simulink model "singlcontact_control_smc_lqr_mydimes_reaction"  (R2024a)
settings: Solver=VariableStepAuto  StartTime=0.0  StopTime=10  FixedStep=0.001  RelTol=1e-3
values from neighbouring files (symbols this model uses):
  ankle_servo_kd = 8    [robotParametersCtrl_mydiem_block_zmp.m]    (also in robotParametersCtrl_quad_modify_mydiem.m; robotParametersCtrl_quad_modify_mydiem_reaction.m)
  ankle_servo_ki = 4    [robotParametersCtrl_mydiem_block_zmp.m]    (also in robotParametersCtrl_quad_modify_mydiem.m; robotParametersCtrl_quad_modify_mydiem_reaction.m)
  ankle_servo_kp = 20    [robotParametersCtrl_mydiem_block_zmp.m]    (also in robotParametersCtrl_quad_modify_mydiem.m; robotParametersCtrl_quad_modify_mydiem_reaction.m)
  deriv_filter_coeff = 100    [robotParametersCtrl_mydiem_block_zmp.m]    (also in robotParametersCtrl_quad_modify_mydiem.m; robotParametersCtrl_quad_modify_mydiem_reaction.m)
  filter_coefficent_pid = 100    [robotParametersCtrl_mydiem_block_zmp.m]    (also in robotParametersCtrl_quad_modify_mydiem.m; robotParametersCtrl_quad_modify_mydiem_reaction.m)
  filter_coefficent_pids = 100    [robotParametersCtrl_quad_modify_mydiem_reaction.m]
  foot_z = 1.5    [robotParametersCtrl_mydiem_block_zmp.m]    (also in robotParametersCtrl_quad_modify_mydiem.m; robotParametersCtrl_quad_modify_mydiem_reaction.m)
  g = 9.81    [ABCDvalues_lqr_quad_mydime_reaction.m]    (also in robotParametersCtrl_mydiem_block_zmp.m = 9.80665; robotParametersCtrl_quad_modify_mydiem.m = 9.80665; robotParametersCtrl_quad_modify_mydiem_reaction.m = 9.80665)
  h = 32    [robotParametersCtrl_mydiem_block_zmp.m]    (also in robotParametersCtrl_quad_modify_mydiem.m; robotParametersCtrl_quad_modify_mydiem_reaction.m)
  height_plane = 0.025    [robotParametersCtrl_mydiem_block_zmp.m]    (also in robotParametersCtrl_quad_modify_mydiem.m; robotParametersCtrl_quad_modify_mydiem_reaction.m)
  hip_pitch_deriv = 20    [robotParametersCtrl_mydiem_block_zmp.m]    (also in robotParametersCtrl_quad_modify_mydiem.m = 200; robotParametersCtrl_quad_modify_mydiem_reaction.m = 200)
  hip_pitch_derivs = 200    [robotParametersCtrl_quad_modify_mydiem_reaction.m]
  hip_pitch_int = 0    [robotParametersCtrl_mydiem_block_zmp.m]    (also in robotParametersCtrl_quad_modify_mydiem.m = 150; robotParametersCtrl_quad_modify_mydiem_reaction.m = 150)
  hip_pitch_ints = 1500    [robotParametersCtrl_quad_modify_mydiem_reaction.m]
  hip_pitch_prop = 10    [robotParametersCtrl_mydiem_block_zmp.m]    (also in robotParametersCtrl_quad_modify_mydiem.m = 500; robotParametersCtrl_quad_modify_mydiem_reaction.m = 500)
  hip_pitch_props = 500    [robotParametersCtrl_quad_modify_mydiem_reaction.m]
  hip_roll_deriv = 28    [robotParametersCtrl_mydiem_block_zmp.m]    (also in robotParametersCtrl_quad_modify_mydiem.m = 280; robotParametersCtrl_quad_modify_mydiem_reaction.m = 280)
  hip_roll_derivs = 280    [robotParametersCtrl_quad_modify_mydiem_reaction.m]
  hip_roll_int = 0    [robotParametersCtrl_mydiem_block_zmp.m]    (also in robotParametersCtrl_quad_modify_mydiem.m = 180; robotParametersCtrl_quad_modify_mydiem_reaction.m = 180)
  hip_roll_ints = 180    [robotParametersCtrl_quad_modify_mydiem_reaction.m]
  hip_roll_prop = 10    [robotParametersCtrl_mydiem_block_zmp.m]    (also in robotParametersCtrl_quad_modify_mydiem.m = 300; robotParametersCtrl_quad_modify_mydiem_reaction.m = 300)
  hip_roll_props = 300    [robotParametersCtrl_quad_modify_mydiem_reaction.m]
  hip_servo_kd = 20    [robotParametersCtrl_mydiem_block_zmp.m]    (also in robotParametersCtrl_quad_modify_mydiem.m; robotParametersCtrl_quad_modify_mydiem_reaction.m)
  hip_servo_ki = 10    [robotParametersCtrl_mydiem_block_zmp.m]    (also in robotParametersCtrl_quad_modify_mydiem.m; robotParametersCtrl_quad_modify_mydiem_reaction.m)
  hip_servo_kp = 60    [robotParametersCtrl_mydiem_block_zmp.m]    (also in robotParametersCtrl_quad_modify_mydiem.m; robotParametersCtrl_quad_modify_mydiem_reaction.m)
  hip_smc_lamda = 85    [robotParametersCtrl_mydiem_block_zmp.m]    (also in robotParametersCtrl_quad_modify_mydiem.m; robotParametersCtrl_quad_modify_mydiem_reaction.m = 95)
  hip_smc_lamdas = 85    [robotParametersCtrl_quad_modify_mydiem_reaction.m]
  hip_smc_new = 25    [robotParametersCtrl_mydiem_block_zmp.m]    (also in robotParametersCtrl_quad_modify_mydiem.m; robotParametersCtrl_quad_modify_mydiem_reaction.m = 45)
  hip_smc_news = 25    [robotParametersCtrl_quad_modify_mydiem_reaction.m]
  init_angs_L = init_angs_R    [robotParametersCtrl_mydiem_block_zmp.m]    (also in robotParametersCtrl_quad_modify_mydiem.m; robotParametersCtrl_quad_modify_mydiem_reaction.m)
  init_angs_R = [0 -sum(init_angs) init_angs(2) 0 init_angs(1)]    [robotParametersCtrl_mydiem_block_zmp.m]    (also in robotParametersCtrl_quad_modify_mydiem.m; robotParametersCtrl_quad_modify_mydiem_reaction.m)
  init_height = h +                torso_z/2 + torso_offset_z + height_plane/2    (= 39.5125)    [robotParametersCtrl_mydiem_block_zmp.m]    (also in robotParametersCtrl_quad_modify_mydiem.m; robotParametersCtrl_quad_modify_mydiem_reaction.m)
  K = lqr(A, B, Q, R)    [ABCDvalues_lqr_quad_mydime_reaction.m]
  knee_pitch_deriv = 10    [robotParametersCtrl_mydiem_block_zmp.m]    (also in robotParametersCtrl_quad_modify_mydiem.m = 100; robotParametersCtrl_quad_modify_mydiem_reaction.m = 100)
  knee_pitch_derivs = 180    [robotParametersCtrl_quad_modify_mydiem_reaction.m]
  knee_pitch_int = 0    [robotParametersCtrl_mydiem_block_zmp.m]    (also in robotParametersCtrl_quad_modify_mydiem.m = 300; robotParametersCtrl_quad_modify_mydiem_reaction.m = 300)
  knee_pitch_ints = 7500    [robotParametersCtrl_quad_modify_mydiem_reaction.m]
  knee_pitch_prop = 10    [robotParametersCtrl_mydiem_block_zmp.m]    (also in robotParametersCtrl_quad_modify_mydiem.m = 400; robotParametersCtrl_quad_modify_mydiem_reaction.m = 400)
  knee_pitch_props = 1200    [robotParametersCtrl_quad_modify_mydiem_reaction.m]
  knee_servo_kd = 10    [robotParametersCtrl_mydiem_block_zmp.m]    (also in robotParametersCtrl_quad_modify_mydiem.m; robotParametersCtrl_quad_modify_mydiem_reaction.m)
  knee_servo_ki = 5    [robotParametersCtrl_mydiem_block_zmp.m]    (also in robotParametersCtrl_quad_modify_mydiem.m; robotParametersCtrl_quad_modify_mydiem_reaction.m)
  knee_servo_kp = 60    [robotParametersCtrl_mydiem_block_zmp.m]    (also in robotParametersCtrl_quad_modify_mydiem.m; robotParametersCtrl_quad_modify_mydiem_reaction.m)
  knee_smc_lamda = 140    [robotParametersCtrl_mydiem_block_zmp.m]    (also in robotParametersCtrl_quad_modify_mydiem.m; robotParametersCtrl_quad_modify_mydiem_reaction.m = 150)
  knee_smc_lamdas = 100    [robotParametersCtrl_quad_modify_mydiem_reaction.m]
  knee_smc_new = 80    [robotParametersCtrl_mydiem_block_zmp.m]    (also in robotParametersCtrl_quad_modify_mydiem.m; robotParametersCtrl_quad_modify_mydiem_reaction.m)
  knee_smc_news = 60    [robotParametersCtrl_quad_modify_mydiem_reaction.m]
  Kwalk = 0.6    [robotParametersCtrl_mydiem_block_zmp.m]    (also in robotParametersCtrl_quad_modify_mydiem.m; robotParametersCtrl_quad_modify_mydiem_reaction.m)
  l1 = 0.20    (= 0.2)    [ABCDvalues_lqr_quad_mydime_reaction.m]
  l2 = 0.20    (= 0.2)    [ABCDvalues_lqr_quad_mydime_reaction.m]
  lower_leg_length = 20    [robotParametersCtrl_mydiem_block_zmp.m]    (also in robotParametersCtrl_quad_modify_mydiem.m; robotParametersCtrl_quad_modify_mydiem_reaction.m)
  m1 = 0.45    [ABCDvalues_lqr_quad_mydime_reaction.m]
  m2 = 0.065    [ABCDvalues_lqr_quad_mydime_reaction.m]
  max_torque = 20    [robotParametersCtrl_mydiem_block_zmp.m]    (also in robotParametersCtrl_quad_modify_mydiem.m; robotParametersCtrl_quad_modify_mydiem_reaction.m)
  motion_time_constant = 0.01    [robotParametersCtrl_mydiem_block_zmp.m]    (also in robotParametersCtrl_quad_modify_mydiem.m; robotParametersCtrl_quad_modify_mydiem_reaction.m)
  plane_x = 25    [robotParametersCtrl_mydiem_block_zmp.m]    (also in robotParametersCtrl_quad_modify_mydiem.m; robotParametersCtrl_quad_modify_mydiem_reaction.m)
  plane_y = 3    [robotParametersCtrl_mydiem_block_zmp.m]    (also in robotParametersCtrl_quad_modify_mydiem.m; robotParametersCtrl_quad_modify_mydiem_reaction.m)
  stepHeight = 0.4    [ABCDvalues_lqr_quad_mydime_reaction.m]
  torso_offset_x = 17    [robotParametersCtrl_mydiem_block_zmp.m]    (also in robotParametersCtrl_quad_modify_mydiem.m; robotParametersCtrl_quad_modify_mydiem_reaction.m)
  torso_offset_x1 = -17    [robotParametersCtrl_mydiem_block_zmp.m]    (also in robotParametersCtrl_quad_modify_mydiem.m; robotParametersCtrl_quad_modify_mydiem_reaction.m)
  torso_offset_z = 0    [robotParametersCtrl_mydiem_block_zmp.m]    (also in robotParametersCtrl_quad_modify_mydiem.m; robotParametersCtrl_quad_modify_mydiem_reaction.m)
  torso_x = 40    [robotParametersCtrl_mydiem_block_zmp.m]    (also in robotParametersCtrl_quad_modify_mydiem.m; robotParametersCtrl_quad_modify_mydiem_reaction.m)
  torso_y = 20    [robotParametersCtrl_mydiem_block_zmp.m]    (also in robotParametersCtrl_quad_modify_mydiem.m; robotParametersCtrl_quad_modify_mydiem_reaction.m)
  torso_z = 15    [robotParametersCtrl_mydiem_block_zmp.m]    (also in robotParametersCtrl_quad_modify_mydiem.m; robotParametersCtrl_quad_modify_mydiem_reaction.m)
  Ts = 0.05    [ABCDvalues_lqr_quad_mydime_reaction.m]
  TsCtrl = 0.05    [robotParametersCtrl_mydiem_block_zmp.m]    (also in robotParametersCtrl_quad_modify_mydiem.m; robotParametersCtrl_quad_modify_mydiem_reaction.m)
  tWalk = 0.3    [robotParametersCtrl_mydiem_block_zmp.m]    (also in robotParametersCtrl_quad_modify_mydiem.m; robotParametersCtrl_quad_modify_mydiem_reaction.m)
  upper_leg_length = 20    [robotParametersCtrl_mydiem_block_zmp.m]    (also in robotParametersCtrl_quad_modify_mydiem.m; robotParametersCtrl_quad_modify_mydiem_reaction.m)
undefined symbols (not defined in the file or in its folder): X, Y, Z
libraries: simulink_extras x256, slpidlib x128, sm_lib x71, simulink x43, nesl_utility x35, walkingRobotUtils x21, dspsrcs4 x18, dspobslib x8
(part 33 of 33)

== system singlcontact_control_smc_lqr_mydimes_reaction/Walking Robot/smc+smcr+neuro1+reaction2/SMC Controllers FR3/Equivalent control/SMC equivalent T1 ==
  theta2 : Inport
  theta1 : Inport  Port=2
  theta2ddot : Inport  Port=3
  theta1dot : Inport  Port=4
  theta2dot : Inport  Port=5
  theta1ddot : Inport  Port=6
  Add{1..4} (4 alike) : Sum
  Add5 : Sum  Inputs=+--+++
  Add6 : Sum  Inputs=++++
  Constant : Constant  Value=0.3
  Constant10 : Constant  Value=m2*l1^2
  Constant11 : Constant  Value=0.3*m1*l1^2
  Constant12 : Constant  Value=m2*l1*l2
  Constant2 : Constant  Value=0.5
  Constant3 : Constant
  Constant4 : Constant  Value=0.5
  Constant5 : Constant
  Constant6 : Constant  Value=g*l1
  Constant7 : Constant  Value=0.5
  Constant9 : Constant  Value=0.3*m2*l2^2
  Cos : Trigonometry  Operator=cos
  Cos1 : Trigonometry  Operator=cos
  Gain1 : Gain  Gain=m2*l2^2
  Gain2 : Gain  Gain=m2*l2*l1
  Gain4 : Gain  Gain=m2*l2*l1
  Gain6 : Gain  Gain=m1
  Gain7 : Gain  Gain=m2
  Gain8 : Gain  Gain=m2*g*l2
  Product{1..3,7..9} (6 alike) : Product
  Product4 : Product  Inputs=4
  Product5 : Product  Inputs=3
  Product6 : Product  Inputs=3
  Sin : Trigonometry
  Sin1 : Trigonometry
  Sin2 : Trigonometry
  Square1 : Math  Operator=square
  T1 : Outport
  wires:
  Add2/1 -> Product1/1
  Product9/1 -> Add2/2
  [lamdaBL1] -> Product9/1
  [edotBL1] -> Product9/2
  Add5/1 -> T1/1
  Product1/1 -> Add5/6
  theta1ddot/1 -> Add2/1
  Add6/1 -> Product1/2
  Product8/1 -> Add6/1
  Constant11/1 -> Add6/2
  Constant10/1 -> Add6/4
  Constant9/1 -> Add6/3
  Cos1/1 -> Product8/1
  Constant12/1 -> Product8/2  "X_dd"
  theta2/1 -> Cos/1, Sin/1, Add4/1, Cos1/1
  Product7/1 -> Add5/5
  Product6/1 -> Add5/4
  Product5/1 -> Add5/3
  Product4/1 -> Add5/2
  Product3/1 -> Add5/1
  Sin2/1 -> Product7/2
  Gain8/1 -> Product7/1
  Add4/1 -> Sin2/1
  Constant7/1 -> Gain8/1
  Constant6/1 -> Product6/3
  Sin1/1 -> Product6/2
  Add3/1 -> Product6/1
  theta1/1 -> Sin1/1, Add4/2
  Gain6/1 -> Add3/1
  Gain7/1 -> Add3/2
  Constant5/1 -> Gain7/1
  Constant4/1 -> Gain6/1
  Square1/1 -> Product5/3
  Constant3/1 -> Gain4/1
  Gain4/1 -> Product4/1
  Sin/1 -> Product5/2, Product4/2
  theta2dot/1 -> Square1/1, Product4/4
  theta1dot/1 -> Product4/3
  Add1/1 -> Product3/2
  theta2ddot/1 -> Product3/1
  Product2/1 -> Add1/2
  Gain1/1 -> Add1/1
  Gain2/1 -> Product5/1, Product2/1
  Cos/1 -> Product2/2
  Constant2/1 -> Gain2/1
  Constant/1 -> Gain1/1

== system singlcontact_control_smc_lqr_mydimes_reaction/Walking Robot/smc+smcr+neuro1+reaction2/SMC Controllers FR3/Equivalent control/SMC equivalent T2 ==
  theta1ddot : Inport
  theta2 : Inport  Port=2
  theta1 : Inport  Port=3
  theta2ddot : Inport  Port=4
  theta1dot : Inport  Port=5
  Add1 : Sum
  Add2 : Sum
  Add4 : Sum
  Add5 : Sum  Inputs=++++
  Constant : Constant  Value=0.5
  Constant1 : Constant  Value=0.3
  Constant2 : Constant  Value=0.5
  Constant3 : Constant
  Gain10 : Gain  Gain=m2*l2^2
  Gain11 : Gain  Gain=m2*l2
  Gain12 : Gain  Gain=g
  Gain13 : Gain  Gain=(1/3)*(m2*(l2^2))
  Gain5 : Gain  Gain=m2*l1*l2
  Product{1..4,7} (5 alike) : Product
  Product6 : Product  Inputs=3
  Sin : Trigonometry
  Square3 : Math  Operator=square
  Trigonometric Function3 : Trigonometry  Operator=cos
  Trigonometric Function4 : Trigonometry
  T2 : Outport
  wires:
  Product2/1 -> Add5/4
  Gain13/1 -> Product2/1
  Add1/1 -> Product2/2
  Constant3/1 -> Gain13/1
  theta2ddot/1 -> Add1/2
  [edotBL2] -> Product1/1
  [lamdaBL2] -> Product1/2
  Product1/1 -> Add1/1
  Add5/1 -> T2/1
  Product7/1 -> Add5/3
  Product6/1 -> Add5/2
  Product4/1 -> Add5/1
  Add4/1 -> Sin/1
  Sin/1 -> Product7/2
  theta1/1 -> Add4/1
  Gain12/1 -> Product7/1
  Gain11/1 -> Gain12/1
  Constant2/1 -> Gain11/1
  Square3/1 -> Product6/3
  theta1dot/1 -> Square3/1
  Trigonometric Function4/1 -> Product6/2
  Constant1/1 -> Gain10/1
  Constant/1 -> Gain5/1
  theta1ddot/1 -> Product4/1
  Add2/1 -> Product4/2
  Gain10/1 -> Add2/2
  Product3/1 -> Add2/1
  Gain5/1 -> Product6/1, Product3/2
  Trigonometric Function3/1 -> Product3/1
  theta2/1 -> Trigonometric Function4/1, Add4/2, Trigonometric Function3/1

== system singlcontact_control_smc_lqr_mydimes_reaction/Walking Robot/smc+smcr+neuro1+reaction2/SMC Controllers FR4/Equivalent control/SMC equivalent T1 ==
  theta2 : Inport
  theta1 : Inport  Port=2
  theta2ddot : Inport  Port=3
  theta1dot : Inport  Port=4
  theta2dot : Inport  Port=5
  theta1ddot : Inport  Port=6
  Add{1..4} (4 alike) : Sum
  Add5 : Sum  Inputs=+--+++
  Add6 : Sum  Inputs=++++
  Constant : Constant  Value=0.3
  Constant10 : Constant  Value=m2*l1^2
  Constant11 : Constant  Value=0.3*m1*l1^2
  Constant12 : Constant  Value=m2*l1*l2
  Constant2 : Constant  Value=0.5
  Constant3 : Constant
  Constant4 : Constant  Value=0.5
  Constant5 : Constant
  Constant6 : Constant  Value=g*l1
  Constant7 : Constant  Value=0.5
  Constant9 : Constant  Value=0.3*m2*l2^2
  Cos : Trigonometry  Operator=cos
  Cos1 : Trigonometry  Operator=cos
  Gain1 : Gain  Gain=m2*l2^2
  Gain2 : Gain  Gain=m2*l2*l1
  Gain4 : Gain  Gain=m2*l2*l1
  Gain6 : Gain  Gain=m1
  Gain7 : Gain  Gain=m2
  Gain8 : Gain  Gain=m2*g*l2
  Product{1..3,7..9} (6 alike) : Product
  Product4 : Product  Inputs=4
  Product5 : Product  Inputs=3
  Product6 : Product  Inputs=3
  Sin : Trigonometry
  Sin1 : Trigonometry
  Sin2 : Trigonometry
  Square1 : Math  Operator=square
  T1 : Outport
  wires:
  Constant/1 -> Gain1/1
  Constant2/1 -> Gain2/1
  Cos/1 -> Product2/2
  Gain2/1 -> Product2/1, Product5/1
  Gain1/1 -> Add1/1
  Product2/1 -> Add1/2
  theta2ddot/1 -> Product3/1
  Add1/1 -> Product3/2
  theta1dot/1 -> Product4/3
  theta2dot/1 -> Product4/4, Square1/1
  Sin/1 -> Product4/2, Product5/2
  Gain4/1 -> Product4/1
  Constant3/1 -> Gain4/1
  Square1/1 -> Product5/3
  Constant4/1 -> Gain6/1
  Constant5/1 -> Gain7/1
  Gain7/1 -> Add3/2
  Gain6/1 -> Add3/1
  theta1/1 -> Add4/2, Sin1/1
  Add3/1 -> Product6/1
  Sin1/1 -> Product6/2
  Constant6/1 -> Product6/3
  Constant7/1 -> Gain8/1
  Add4/1 -> Sin2/1
  Gain8/1 -> Product7/1
  Sin2/1 -> Product7/2
  Product3/1 -> Add5/1
  Product4/1 -> Add5/2
  Product5/1 -> Add5/3
  Product6/1 -> Add5/4
  Product7/1 -> Add5/5
  theta2/1 -> Cos1/1, Add4/1, Sin/1, Cos/1
  Constant12/1 -> Product8/2  "X_dd"
  Cos1/1 -> Product8/1
  Constant9/1 -> Add6/3
  Constant10/1 -> Add6/4
  Constant11/1 -> Add6/2
  Product8/1 -> Add6/1
  Add6/1 -> Product1/2
  theta1ddot/1 -> Add2/1
  Product1/1 -> Add5/6
  Add5/1 -> T1/1
  [edotFR1s] -> Product9/2
  [lamdaFR1s] -> Product9/1
  Product9/1 -> Add2/2
  Add2/1 -> Product1/1

== system singlcontact_control_smc_lqr_mydimes_reaction/Walking Robot/smc+smcr+neuro1+reaction2/SMC Controllers FR4/Equivalent control/SMC equivalent T2 ==
  theta1ddot : Inport
  theta2 : Inport  Port=2
  theta1 : Inport  Port=3
  theta2ddot : Inport  Port=4
  theta1dot : Inport  Port=5
  Add1 : Sum
  Add2 : Sum
  Add4 : Sum
  Add5 : Sum  Inputs=++++
  Constant : Constant  Value=0.5
  Constant1 : Constant  Value=0.3
  Constant2 : Constant  Value=0.5
  Constant3 : Constant
  Gain10 : Gain  Gain=m2*l2^2
  Gain11 : Gain  Gain=m2*l2
  Gain12 : Gain  Gain=g
  Gain13 : Gain  Gain=(1/3)*(m2*(l2^2))
  Gain5 : Gain  Gain=m2*l1*l2
  Product{1..4,7} (5 alike) : Product
  Product6 : Product  Inputs=3
  Sin : Trigonometry
  Square3 : Math  Operator=square
  Trigonometric Function3 : Trigonometry  Operator=cos
  Trigonometric Function4 : Trigonometry
  T2 : Outport
  wires:
  theta2/1 -> Trigonometric Function3/1, Add4/2, Trigonometric Function4/1
  Trigonometric Function3/1 -> Product3/1
  Gain5/1 -> Product3/2, Product6/1
  Product3/1 -> Add2/1
  Gain10/1 -> Add2/2
  Add2/1 -> Product4/2
  theta1ddot/1 -> Product4/1
  Constant/1 -> Gain5/1
  Constant1/1 -> Gain10/1
  Trigonometric Function4/1 -> Product6/2
  theta1dot/1 -> Square3/1
  Square3/1 -> Product6/3
  Constant2/1 -> Gain11/1
  Gain11/1 -> Gain12/1
  Gain12/1 -> Product7/1
  theta1/1 -> Add4/1
  Sin/1 -> Product7/2
  Add4/1 -> Sin/1
  Product4/1 -> Add5/1
  Product6/1 -> Add5/2
  Product7/1 -> Add5/3
  Add5/1 -> T2/1
  Product1/1 -> Add1/1
  [lamdaFR2s] -> Product1/2
  [edotFR2s] -> Product1/1
  theta2ddot/1 -> Add1/2
  Constant3/1 -> Gain13/1
  Add1/1 -> Product2/2
  Gain13/1 -> Product2/1
  Product2/1 -> Add5/4

== matlab function singlcontact_control_smc_lqr_mydimes_reaction/Walking Controller/ZMP Controller/Log Step Lengths/MATLAB Function ==
  data: input input; y output; in_rate input; out_rate input
function y = zeroOrderHold(input, in_rate, out_rate)
    persistent buffer;
    persistent counter;

    if nargin < 3
        error('Input and output rates must be specified.');
    end

    if isempty(buffer)
        buffer = input;
        counter = 1;
        y = zeros(size(input)); % Initialize y to be the same size as input
    else
        buffer = [buffer; input];
        counter = counter + 1;
    end
    
    if counter == ceil(out_rate / in_rate) || isempty(input)
        y = buffer(1,:);
        buffer = buffer(2:end,:);
        counter = 1;
    else
        y = buffer(1,:);
    end
end

== stateflow chart singlcontact_control_smc_lqr_mydimes_reaction/Walking Controller/Step Planning Logic ==
  settings: updateMethod=DISCRETE  sampleTime=TsCtrl
  state control [function]
    (default) -> (junction 43) : {
        | xR = xR + Kwalk*(xrefR-xR);
        | yR = yR + Kwalk*(yrefR-yR);
        | zR = zR + Kwalk*(zrefR-zR);
        | xL = xL + Kwalk*(xrefL-xL);
        | yL = yL + Kwalk*(yrefL-yL);
        | zL = zL + Kwalk*(zrefL-zL);
        | footR = [xR;yR;zR];
        | footL = [xL;yL;zL];
        | }
  state LeftStep
    % Left foot is active
    % Right foot drags
    en, du:
    control;
    state RightFoot [parallel]
      en,du:
      xrefR = -xrefL;
      yrefR = -max(0,stepLat);
      settings: executionOrder=2
    state LeftFoot [parallel]
      en,du:
      zrefR = low;
      xrefL = stepFwd;
      yrefL = max(0,stepLat);
      zrefL = high;
      on after(0.5*tWalk,sec):
      zrefL = low;
      settings: executionOrder=1
  state RightStep
    % Right foot is active
    % Left foot drags
    en, du:
    control;
    state RightFoot [parallel]
      en,du:
      zrefL = low;
      xrefR = stepFwd;
      yrefR = min(0,stepLat);
      zrefR = high;
      on after(0.5*tWalk,sec):
      zrefR = low;
      settings: executionOrder=1
    state LeftFoot [parallel]
      en,du:
      xrefL = -xrefR;
      yrefL = -min(stepLat,0);
      settings: executionOrder=2
  (default) -> RightStep : % Initialize values
      | {
      | low = -h/100;
      | high = low + stepHeight;
      | xL = 0; yL = 0; zL = low;
      | xR = 0; yR = 0; zR = low;
      | xrefL = 0; yrefL = 0; zrefL = low;
      | xrefR = 0; yrefR = 0; zrefR = low;
      | }
  RightStep -> LeftStep : [after(tWalk,sec)]
  LeftStep -> RightStep : [after(tWalk,sec)]
  data: footR output; footL output; stepFwd input; stepLat input; xR local; yR local; zR local; high local; xL local; yL local; zL local; low local; stepHeight parameter; h parameter; Kwalk parameter; yrefL local; zrefL local; xrefL local; yrefR local; zrefR local; xrefR local; tWalk parameter

== matlab function singlcontact_control_smc_lqr_mydimes_reaction/Walking Controller/ZMP Controller/MATLAB Function3 ==
  data: Xref input; posoutx output; Yref input; Xmes input; posouty output; Ymes input; accel_x input; accel_y input; R input
function [ posoutx, posouty] = footsteps_Right_Left_modified_test_acc(Xref, Yref,Xmes,Ymes,accel_x,accel_y,R)
    foot_x = 9;
    foot_y = 5;
    in_rate=0;
    out_rate=0.3;
    % 
    % Initialize footR and footL
    low = -32/100; % height is h=94%
    high = low + 0.08; % step height = 0.03%
    % Initialize stepFwd_1 and stepLat_1 as empty matrices
    % stepFwd_1 = [];
    % stepLat_1 = [];

    zrefL = low;
    zrefR = low;
    % 
    % persistent xR yR zR xL yL zL;
    % if isempty(xR)
    %     xR = 0; yR = 0; zR = low;
    %     xL = 0; yL = 0; zL = low;
    % end

    persistent errXm errYm last_ax_glob last_ay_glob;
    if isempty(errXm)
        errXm = 0;
        errYm = 0;
        last_ax_glob = 0; % Initialize last_ax_glob
        last_ay_glob = 0; % Initialize last_ay_glob
    end

    %% PID gains% for smc%%
    xKp = 8.5;
    xKi = 0;
    xKd = 0.01;
    yKp =4;
    yKi = 0;
    yKd = 0.1;

    % % PID gains for pid %%
    % xKp = 1;
    % xKi = 0;
    % xKd = 0;
    % yKp =1;
    % yKi = 0;
    % yKd = 0;
    

    % Error calculations
    errX = Xref - Xmes;
    errY = Yref - Ymes;

    % % Error calculations
    % errX = Xref - Xref;
    % errY = Yref - Yref;

    % Calculate control signals with filtering in derivative term
    N = 0.5; % Filter coefficient (adjust as needed)
    ax_glob = xKp * errX + ((xKd * errX) - errXm) * N + (1 - N) * last_ax_glob;
    ay_glob = yKp * errY + ((yKd * errY) - errYm) * N + (1 - N) * last_ay_glob;

    % % Update error memory
    errXm = (errXm + errX) * 0.05;
    errYm = (errYm + errY) * 0.05;

    % Update last control signals for filtering
    last_ax_glob = ax_glob;
    last_ay_glob = ay_glob;

    % Additional constant and matrix operations
    az_glob = 0;

    % Debugging: Print the values of ax_glob and ay_glob
    % disp(['Values of az_glob: ', num2str(az_glob)]);

    % % Ensure that ax_glob, ay_glob, and az_glob are scalars
    % ax_glob = scalarCheck(ax_glob);
    % ay_glob = scalarCheck(ay_glob);
    % az_glob = scalarCheck(az_glob);

    control_matrix = [ax_glob; ay_glob; az_glob];
    % % disp([ax_glob; ay_glob; az_glob])
    % 
    % % Transpose R matrix and perform matrix multiplication
    a_loc = (R)' * control_matrix;

    % Multiplication with the provided expression
    g = 9.81;
    h_minus_torso_offset_z = 32;
    posin = a_loc * ((h_minus_torso_offset_z) / (g * 100));
  
    % % Form the acceleration matrix and multiply with R transpose
    acceleration_matrix = [accel_x; accel_y; 0];
    a_loc2 = (R)' * acceleration_matrix;

    % Multiply with the provided expression
    a_loc2_modified = a_loc2 * ((h_minus_torso_offset_z) / (g * 100));
    

    posinx= posin(1, :);
    posiny= posin(2, :);

    a_loc2_modifiedx=a_loc2_modified(1, :);
    a_loc2_modifiedy=a_loc2_modified(2, :);

    % Call saturationBlock for posoutx
    posoutx = saturationBlock((0.9 * ((foot_x / 2) / 100 )+ a_loc2_modified(1, :)), posin(1, :), (-0.9 * ((foot_x / 2) / 100) + a_loc2_modified(1, :)));

    % Call saturationBlock for posouty
    posouty = saturationBlock((0.9 * ((foot_y / 2) / 100) + a_loc2_modified(2, :)), posin(2, :), (-0.9 * ((foot_x / 2) / 100) + a_loc2_modified(2, :)));
    % % Call saturationBlock for posoutx
    % posoutx = saturationBlock((a_loc2_modified(1, :)), posin(1, :), a_loc2_modified(1, :));
    % 
    % % Call saturationBlock for posouty
    % posouty = saturationBlock((a_loc2_modified(2, :)), posin(2, :), a_loc2_modified(2, :));


    % % % Obtain stepFwd and stepLat from zeroOrderHold function using the current time (k)
    % stepFwd = zeroOrderHold(posoutx, 0, 0.3);
    % stepLat = zeroOrderHold(posouty, 0, 0.3);
    % 
    % % % Specify the size of the output as variable-size
    % % stepFwd_1 = zeros(1,1); % Initialize as a scalar
    % % stepLat_1 = zeros(1,1); % Initialize as a scalar
    % 
    % % Obtain stepFwd and stepLat from zeroOrderHold function using the current time (k)
    % stepFwd_1 = stepFwd *100;
    % stepLat_1 = stepLat *100;

%     if (rem(fix(i / 6), 2) == 0)
%         [footR, footL] = stateflowRL(stepFwd_1, stepLat_1, i, xL, yL, zL, xR, yR, zR, xrefL, yrefL, zrefL, xrefR, yrefR, zrefR, low, high); %right foot
% else
%         [footR, footL] = stateflowLR(stepFwd_1, stepLat_1, i, xL, yL, zL, xR, yR, zR, xrefL, yrefL, zrefL, xrefR, yrefR, zrefR, low, high); %left foot
%     end
end

function output = saturationBlock(input1, input2, input3)
    % Define lower and upper limits
    lower_limit = input3; % Define lower limit
    upper_limit = input1;  % Define upper limit

    % Calculate output
    output = min(upper_limit, max(lower_limit, input2));

    % % Ensure output type is integer and rounding mode is floor
    % output = floor(output);
end


% function y = zeroOrderHold(input, in_rate, out_rate)
%     persistent buffer;
%     persistent counter;
% 
%     if nargin < 3
%         error('Input and output rates must be specified.');
%     end
% 
%     if isempty(buffer)
%         buffer = input;
%         counter = 1;
%         y = zeros(size(input)); % Initialize y to be the same size as input
%     else
%         buffer = [buffer; input];
%         counter = counter + 1;
%     end
% 
%     if counter == ceil(out_rate / in_rate) || isempty(input)
%         y = buffer(1,:);
%         buffer = buffer(2:end,:);
%         counter = 1;
%     else
%         y = buffer(1,:);
%     end
% end

== matlab function singlcontact_control_smc_lqr_mydimes_reaction/Walking Controller/ZMP Controller/Log Step Lengths/MATLAB Function1 ==
  data: input input; y output; in_rate input; out_rate input
function y = zeroOrderHold(input, in_rate, out_rate)
    persistent buffer;
    persistent counter;

    if nargin < 3
        error('Input and output rates must be specified.');
    end

    if isempty(buffer)
        buffer = input;
        counter = 1;
        y = zeros(size(input)); % Initialize y to be the same size as input
    else
        buffer = [buffer; input];
        counter = counter + 1;
    end
    
    if counter == ceil(out_rate / in_rate) || isempty(input)
        y = buffer(1,:);
        buffer = buffer(2:end,:);
        counter = 1;
    else
        y = buffer(1,:);
    end
end

== matlab function singlcontact_control_smc_lqr_mydimes_reaction/Walking Controller/ZMP Controller/MATLAB Function1 ==
  data: Xref input; posoutFRx output; Yref input; Xmes input; Ymes input; accel_x input; accel_y input; posoutFRy output; R input; posoutFLx output; posoutFLy output; posoutBRx output; posoutBRy output; posoutBLx output; posoutBLy output
function [ posoutFRx, posoutFRy, posoutFLx, posoutFLy, posoutBRx, posoutBRy, posoutBLx, posoutBLy ] = footsteps_Quadruped(Xref, Yref, Xmes, Ymes, accel_x, accel_y, R)
    % Initialize foot positions and step parameters for all four legs
    foot_x = 5;
    foot_y = 4;
    in_rate = 0;
    out_rate = 0.3;
    low = -18/100;
    high = low + 0.02;

    % Initialize persistent variables for errors and last control signals
    persistent errXmFR errYmFR errXmFL errYmFL errXmBR errYmBR errXmBL errYmBL;
    persistent last_ax_globFR last_ay_globFR last_ax_globFL last_ay_globFL;
    persistent last_ax_globBR last_ay_globBR last_ax_globBL last_ay_globBL;

    if isempty(errXmFR)
        errXmFR = 0; errYmFR = 0; last_ax_globFR = 0; last_ay_globFR = 0;
        errXmFL = 0; errYmFL = 0; last_ax_globFL = 0; last_ay_globFL = 0;
        errXmBR = 0; errYmBR = 0; last_ax_globBR = 0; last_ay_globBR = 0;
        errXmBL = 0; errYmBL = 0; last_ax_globBL = 0; last_ay_globBL = 0;
    end

    % PID gains
    Kp = 20; Ki = 0; Kd = 2.5;
    N = 0.5; % Filter coefficient

    % Calculate errors
    errXFR = Xref - Xmes; errYFR = Yref - Ymes;
    errXFL = Xref - Xmes; errYFL = Yref - Ymes;
    errXBR = Xref - Xmes; errYBR = Yref - Ymes;
    errXBL = Xref - Xmes; errYBL = Yref - Ymes;

    % Control signals with filtering in derivative term
    ax_globFR = Kp * errXFR + ((Kd * errXFR) - errXmFR) * N + (1 - N) * last_ax_globFR;
    ay_globFR = Kp * errYFR + ((Kd * errYFR) - errYmFR) * N + (1 - N) * last_ay_globFR;
    ax_globFL = Kp * errXFL + ((Kd * errXFL) - errXmFL) * N + (1 - N) * last_ax_globFL;
    ay_globFL = Kp * errYFL + ((Kd * errYFL) - errYmFL) * N + (1 - N) * last_ay_globFL;
    ax_globBR = Kp * errXBR + ((Kd * errXBR) - errXmBR) * N + (1 - N) * last_ax_globBR;
    ay_globBR = Kp * errYBR + ((Kd * errYBR) - errYmBR) * N + (1 - N) * last_ay_globBR;
    ax_globBL = Kp * errXBL + ((Kd * errXBL) - errXmBL) * N + (1 - N) * last_ax_globBL;
    ay_globBL = Kp * errYBL + ((Kd * errYBL) - errYmBL) * N + (1 - N) * last_ay_globBL;

    % Update error memory
    errXmFR = (errXmFR + errXFR) * 0.05;
    errYmFR = (errYmFR + errYFR) * 0.05;
    errXmFL = (errXmFL + errXFL) * 0.05;
    errYmFL = (errYmFL + errYFL) * 0.05;
    errXmBR = (errXmBR + errXBR) * 0.05;
    errYmBR = (errYmBR + errYBR) * 0.05;
    errXmBL = (errXmBL + errXBL) * 0.05;
    errYmBL = (errYmBL + errYBL) * 0.05;

    % Update last control signals for filtering
    last_ax_globFR = ax_globFR;
    last_ay_globFR = ay_globFR;
    last_ax_globFL = ax_globFL;
    last_ay_globFL = ay_globFL;
    last_ax_globBR = ax_globBR;
    last_ay_globBR = ay_globBR;
    last_ax_globBL = ax_globBL;
    last_ay_globBL = ay_globBL;

    % Coordinate transformation and position calculation
    az_glob = 0;
    control_matrix_FR = [ax_globFR; ay_globFR; az_glob];
    control_matrix_FL = [ax_globFL; ay_globFL; az_glob];
    control_matrix_BR = [ax_globBR; ay_globBR; az_glob];
    control_matrix_BL = [ax_globBL; ay_globBL; az_glob];

    a_loc_FR = (R)' * control_matrix_FR;
    a_loc_FL = (R)' * control_matrix_FL;
    a_loc_BR = (R)' * control_matrix_BR;
    a_loc_BL = (R)' * control_matrix_BL;

    g = 9.81;
    h_minus_torso_offset_z = 20;

    posin_FR = a_loc_FR * ((h_minus_torso_offset_z) / (g * 100));
    posin_FL = a_loc_FL * ((h_minus_torso_offset_z) / (g * 100));
    posin_BR = a_loc_BR * ((h_minus_torso_offset_z) / (g * 100));
    posin_BL = a_loc_BL * ((h_minus_torso_offset_z) / (g * 100));

    % Acceleration adjustment
    acceleration_matrix = [accel_x; accel_y; 0];
    a_loc2_FR = (R)' * acceleration_matrix;
    a_loc2_FL = (R)' * acceleration_matrix;
    a_loc2_BR = (R)' * acceleration_matrix;
    a_loc2_BL = (R)' * acceleration_matrix;

    a_loc2_modified_FR = a_loc2_FR * ((h_minus_torso_offset_z) / (g * 100));
    a_loc2_modified_FL = a_loc2_FL * ((h_minus_torso_offset_z) / (g * 100));
    a_loc2_modified_BR = a_loc2_BR * ((h_minus_torso_offset_z) / (g * 100));
    a_loc2_modified_BL = a_loc2_BL * ((h_minus_torso_offset_z) / (g * 100));

    % Calculate desired foot positions and apply saturation
    posoutFRx = saturationBlock((0.9 * (foot_x / 2) / 100 + a_loc2_modified_FR(1, :)), posin_FR(1, :), (-0.9 * (foot_x / 2) / 100 + a_loc2_modified_FR(1, :)));
    posoutFRy = saturationBlock((0.9 * ((foot_y / 2) / 100) + a_loc2_modified_FR(2, :)), posin_FR(2, :), (-0.9 * ((foot_x / 2) / 100) + a_loc2_modified_FR(2, :)));

    posoutFLx = saturationBlock((0.9 * (foot_x / 2) / 100 + a_loc2_modified_FL(1, :)), posin_FL(1, :), (-0.9 * (foot_x / 2) / 100 + a_loc2_modified_FL(1, :)));
    posoutFLy = saturationBlock((0.9 * ((foot_y / 2) / 100) + a_loc2_modified_FL(2, :)), posin_FL(2, :), (-0.9 * ((foot_x / 2) / 100) + a_loc2_modified_FL(2, :)));

    posoutBRx = saturationBlock((0.9 * (foot_x / 2) / 100 + a_loc2_modified_BR(1, :)), posin_BR(1, :), (-0.9 * (foot_x / 2) / 100 + a_loc2_modified_BR(1, :)));
    posoutBRy = saturationBlock((0.9 * ((foot_y / 2) / 100) + a_loc2_modified_BR(2, :)), posin_BR(2, :), (-0.9 * ((foot_x / 2) / 100) + a_loc2_modified_BR(2, :)));

    posoutBLx = saturationBlock((0.9 * (foot_x / 2) / 100 + a_loc2_modified_BL(1, :)), posin_BL(1, :), (-0.9 * (foot_x / 2) / 100 + a_loc2_modified_BL(1, :)));
    posoutBLy = saturationBlock((0.9 * ((foot_y / 2) / 100) + a_loc2_modified_BL(2, :)), posin_BL(2, :), (-0.9 * ((foot_x / 2) / 100) + a_loc2_modified_BL(2, :)));
end

% Helper function to ensure the calculated foot positions stay within bounds
function output = saturationBlock(input1, input2, input3)
    lower_limit = input3;
    upper_limit = input1;
    output = min(upper_limit, max(lower_limit, input2));
end

== matlab function singlcontact_control_smc_lqr_mydimes_reaction/Walking Controller/final logic working quad_walk1 ==
  settings: updateMethod=DISCRETE
  data: stepFwd input; footFR output; stepLat input; timeElapsed input; footFL output; footBR output; footBL output
function [footFR, footFL, footBR, footBL] = stateflow_version_workingfine_walk(stepFwd, stepLat, timeElapsed)
    tWalk = 0.3;        % Walking gait period (s)

Kwalk = 0.5;        % Walking gain for tracking XYZ foot positions

    % Initialize foot positions
    low = -18/100; % Base height
    high = low + 0.02; % Step height

    % Persistent variables to store positions and references
    persistent xFR yFR zFR xFL yFL zFL xBR yBR zBR xBL yBL zBL
    persistent xrefFR yrefFR zrefFR xrefFL yrefFL zrefFL xrefBR yrefBR zrefBR xrefBL yrefBL zrefBL
    persistent lastUpdateTime phase

    % Initialize variables if this is the first call
    if isempty(lastUpdateTime)
        xFR = 0; yFR = 0; zFR = low;
        xFL = 0; yFL = 0; zFL = low;
        xBR = 0; yBR = 0; zBR = low;
        xBL = 0; yBL = 0; zBL = low;
        xrefFR = 0; yrefFR = 0; zrefFR = low;
        xrefFL = 0; yrefFL = 0; zrefFL = low;
        xrefBR = 0; yrefBR = 0; zrefBR = low;
        xrefBL = 0; yrefBL = 0; zrefBL = low;
        lastUpdateTime = 0;
        phase = 0;
    end

    % Calculate the elapsed time since the last update
    deltaTime = timeElapsed - lastUpdateTime;

    % Control logic for walking gait
    switch phase
        case 0 % Move front-left leg
            zrefFL = high;
            xrefFL = stepFwd;
            yrefFL = stepLat;
            zrefFR = low;
            zrefBR = low;
            zrefBL = low;
            if deltaTime > tWalk/4
                phase = 1;
                lastUpdateTime = timeElapsed;
                fprintf('Phase 0 to 1: Front-left leg moves\n');
            end
        case 1 % Move back-right leg
            zrefBR = high;
            xrefBR = stepFwd;
            yrefBR = -stepLat;
            zrefFR = low;
            zrefFL = low;
            zrefBL = low;
            if deltaTime > tWalk/4
                phase = 2;
                lastUpdateTime = timeElapsed;
                fprintf('Phase 1 to 2: Back-right leg moves\n');
            end
        case 2 % Move front-right leg
            zrefFR = high;
            xrefFR = stepFwd;
            yrefFR = -stepLat;
            zrefFL = low;
            zrefBR = low;
            zrefBL = low;
            if deltaTime > tWalk/4
                phase = 3;
                lastUpdateTime = timeElapsed;
                fprintf('Phase 2 to 3: Front-right leg moves\n');
            end
        case 3 % Move back-left leg
            zrefBL = high;
            xrefBL = stepFwd;
            yrefBL = stepLat;
            zrefFR = low;
            zrefFL = low;
            zrefBR = low;
            if deltaTime > tWalk/4
                phase = 0;
                lastUpdateTime = timeElapsed;
                fprintf('Phase 3 to 0: Back-left leg moves\n');
            end
    end

    % Update positions
    xFR = xFR + Kwalk * (xrefFR - xFR);
    yFR = yFR + Kwalk * (yrefFR - yFR);
    zFR = zFR + Kwalk * (zrefFR - zFR);
    xFL = xFL + Kwalk * (xrefFL - xFL);
    yFL = yFL + Kwalk * (yrefFL - yFL);
    zFL = zFL + Kwalk * (zrefFL - zFL);
    xBR = xBR + Kwalk * (xrefBR - xBR);
    yBR = yBR + Kwalk * (yrefBR - yBR);
    zBR = zBR + Kwalk * (zrefBR - zBR);
    xBL = xBL + Kwalk * (xrefBL - xBL);
    yBL = yBL + Kwalk * (yrefBL - yBL);
    zBL = zBL + Kwalk * (zrefBL - zBL);

    % Ensure that foot positions have three rows
    footFR = [xFR; yFR; zFR];
    footFL = [xFL; yFL; zFL];
    footBR = [xBR; yBR; zBR];
    footBL = [xBL; yBL; zBL];

    % Debugging output for foot positions
    fprintf('Foot positions:\n');
    fprintf('FR: [%f, %f, %f]\n', xFR, yFR, zFR);
    fprintf('FL: [%f, %f, %f]\n', xFL, yFL, zFL);
    fprintf('BR: [%f, %f, %f]\n', xBR, yBR, zBR);
    fprintf('BL: [%f, %f, %f]\n', xBL, yBL, zBL);

    % Update last update time
    lastUpdateTime = timeElapsed;
end

== matlab function singlcontact_control_smc_lqr_mydimes_reaction/Walking Controller/final logic working quad_trot ==
  settings: updateMethod=DISCRETE
  data: stepFwd input; footFR output; stepLat input; timeElapsed input; footFL output; footBR output; footBL output
function [footFR, footFL, footBR, footBL] = stateflow_version_workingfine_trot(stepFwd, stepLat, timeElapsed)
    Kwalk = 0.5;
    tWalk = 0.3; % Set the duration of a full walk cycle

    % Initialize foot positions
    low = -32/100; % height is h=94%
    high = low + 0.04; % step height = 0.03%

    % Persistent variables to store positions and references
    persistent xFR yFR zFR xFL yFL zFL xBR yBR zBR xBL yBL zBL
    persistent xrefFR yrefFR zrefFR xrefFL yrefFL zrefFL xrefBR yrefBR zrefBR xrefBL yrefBL zrefBL
    persistent lastUpdateTime

    % Initialize variables if this is the first call
    if isempty(lastUpdateTime)
        xFR = 0; yFR = 0; zFR = low;
        xFL = 0; yFL = 0; zFL = low;
        xBR = 0; yBR = 0; zBR = low;
        xBL = 0; yBL = 0; zBL = low;
        xrefFR = 0; yrefFR = 0; zrefFR = low;
        xrefFL = 0; yrefFL = 0; zrefFL = low;
        xrefBR = 0; yrefBR = 0; zrefBR = low;
        xrefBL = 0; yrefBL = 0; zrefBL = low;
        lastUpdateTime = 0;
    end

    % Calculate the elapsed time since the last update
    deltaTime = timeElapsed - lastUpdateTime;

    % Control logic for alternating legs
    if rem(fix(lastUpdateTime/tWalk), 2) == 0
        % Phase 1: Move FR and BL
        zrefFL = low;
        zrefBR = low;
        xrefFR = stepFwd;
        yrefFR = min(0, stepLat);
        zrefFR = high;
        xrefBL = stepFwd;
        yrefBL = min(0, stepLat);
        zrefBL = high;

        % Ensure feet are low if mid-step
        if rem((ceil(lastUpdateTime/tWalk)), 2) == 1 && rem((ceil(lastUpdateTime/(tWalk/2))), 2) == 0
            zrefFR = low;
            zrefBL = low;
        end

        % Opposite legs static
        xrefFL = -xrefFR;
        yrefFL = -min(stepLat, 0);
        xrefBR = -xrefBL;
        yrefBR = -min(stepLat, 0);
    else
        % Phase 2: Move FL and BR
        zrefFR = low;
        zrefBL = low;
        xrefFL = stepFwd;
        yrefFL = max(0, stepLat);
        zrefFL = high;
        xrefBR = stepFwd;
        yrefBR = max(0, stepLat);
        zrefBR = high;

        % Ensure feet are low if mid-step
        if rem((ceil(lastUpdateTime/tWalk)), 2) == 0 && rem((ceil(lastUpdateTime/(tWalk/2))), 2) == 0
            zrefFL = low;
            zrefBR = low;
        end

         % Opposite legs static
        xrefFR = -xrefFL;
        yrefFR = -max(stepLat, 0);
        xrefBL = -xrefBR;
        yrefBL = -max(stepLat, 0);
    end

    % Update positions
    xFR = xFR + Kwalk * (xrefFR - xFR) %* deltaTime;
    yFR = yFR + Kwalk * (yrefFR - yFR) %* deltaTime;
    zFR = zFR + Kwalk * (zrefFR - zFR) %* deltaTime;
    xFL = xFL + Kwalk * (xrefFL - xFL) %* deltaTime;
    yFL = yFL + Kwalk * (yrefFL - yFL) %* deltaTime;
    zFL = zFL + Kwalk * (zrefFL - zFL) %* deltaTime;
    xBR = xBR + Kwalk * (xrefBR - xBR) %* deltaTime;
    yBR = yBR + Kwalk * (yrefBR - yBR) %* deltaTime;
    zBR = zBR + Kwalk * (zrefBR - zBR) %* deltaTime;
    xBL = xBL + Kwalk * (xrefBL - xBL) %* deltaTime;
    yBL = yBL + Kwalk * (yrefBL - yBL) %* deltaTime;
    zBL = zBL + Kwalk * (zrefBL - zBL) %* deltaTime;

    % Ensure that foot positions have three rows
    footFR = [xFR; yFR; zFR];
    footFL = [xFL; yFL; zFL];
    footBR = [xBR; yBR; zBR];
    footBL = [xBL; yBL; zBL];

    % Update last update time
    lastUpdateTime = timeElapsed;
end

== matlab function singlcontact_control_smc_lqr_mydimes_reaction/Walking Robot/smc+smcr+neuro1+reaction2/MATLAB Function ==
  data: smc_output input; blended_output output; lqr_output input; switch_flag input; transition_rate input
function blended_output = smooth_blend(smc_output, lqr_output, switch_flag, transition_rate)
    % Inputs:
    % smc_output: 3-element vector from SMC (e.g., [knee, hip_roll, hip_pitch])
    % lqr_output: 3-element vector from LQR (e.g., [knee, hip_roll, hip_pitch])
    % switch_flag: Binary signal indicating whether to use SMC (1) or LQR (0)
    % transition_rate: Rate of blending transition (0 to 1 range per step)
    
    % Initialize blended_output as the same size as input vectors
    blended_output = zeros(3, 1);

    % Loop through each joint control element
    for i = 1:3
        % Calculate smooth blend for each element
        blended_output(i) = (1 - transition_rate) * smc_output(i) + transition_rate * lqr_output(i);
    end
    
    % Adjust transition rate based on switch_flag
    if switch_flag == 1
        % When switch_flag is 1, stay closer to SMC output
        transition_rate = max(transition_rate - 0.05, 0);  % Adjust rate as needed
    else
        % When switch_flag is 0, move towards LQR output
        transition_rate = min(transition_rate + 0.05, 1);  % Adjust rate as needed
    end
end

== matlab function singlcontact_control_smc_lqr_mydimes_reaction/Walking Controller/ZMP Controller/original ==
  data: Xref input; posoutx output; Yref input; Xmes input; Ymes input; accel_x input; accel_y input; posouty output; R input
function [posoutx,posouty] = footsteps_Right_Left_modified_test_acc(Xref, Yref,Xmes,Ymes,accel_x,accel_y,R)
    foot_x = 5;
    foot_y = 4;
    % 
    % Initialize footR and footL
    low = -18/100; % height is h=94%
    high = low + 0.02; % step height = 0.03%

    zrefL = low;
    zrefR = low;
    % 
    % persistent xR yR zR xL yL zL;
    % if isempty(xR)
    %     xR = 0; yR = 0; zR = low;
    %     xL = 0; yL = 0; zL = low;
    % end

    persistent errXm errYm last_ax_glob last_ay_glob;
    if isempty(errXm)
        errXm = 0;
        errYm = 0;
        last_ax_glob = 0; % Initialize last_ax_glob
        last_ay_glob = 0; % Initialize last_ay_glob
    end

    % PID gains
    Kp = 20;
    Ki = 0;
    Kd = 2.5;

    % Error calculations
    errX = Xref - Xmes;
    errY = Yref - Ymes;

    % Calculate control signals with filtering in derivative term
    N = 0.5; % Filter coefficient (adjust as needed)
    ax_glob = Kp * errX + ((Kd * errX) - errXm) * N + (1 - N) * last_ax_glob;
    ay_glob = Kp * errY + ((Kd * errY) - errYm) * N + (1 - N) * last_ay_glob;

    % % Update error memory
    errXm = (errXm + errX) * 0.05;
    errYm = (errYm + errY) * 0.05;

    % Update last control signals for filtering
    last_ax_glob = ax_glob;
    last_ay_glob = ay_glob;

    % Additional constant and matrix operations
    az_glob = 0;

    % Debugging: Print the values of ax_glob and ay_glob
    % disp(['Values of az_glob: ', num2str(az_glob)]);

    % % Ensure that ax_glob, ay_glob, and az_glob are scalars
    % ax_glob = scalarCheck(ax_glob);
    % ay_glob = scalarCheck(ay_glob);
    % az_glob = scalarCheck(az_glob);

    control_matrix = [ax_glob; ay_glob; az_glob];
    % % disp([ax_glob; ay_glob; az_glob])
    % 
    % % Transpose R matrix and perform matrix multiplication
    a_loc = (R)' * control_matrix;

    % Multiplication with the provided expression
    g = 9.81;
    h_minus_torso_offset_z = 20;
    posin = a_loc * ((h_minus_torso_offset_z) / (g * 100));
  
    % % Form the acceleration matrix and multiply with R transpose
    acceleration_matrix = [accel_x; accel_y; 0];
    a_loc2 = (R)' * acceleration_matrix;

    % Multiply with the provided expression
    a_loc2_modified = a_loc2 * ((h_minus_torso_offset_z) / (g * 100));
    

    posinx= posin(1, :);
    posiny= posin(2, :);

    a_loc2_modifiedx=a_loc2_modified(1, :);
    a_loc2_modifiedy=a_loc2_modified(2, :);

    % Call saturationBlock for posoutx
    posoutx = saturationBlock((0.9 * (foot_x / 2) / 100 + a_loc2_modified(1, :)), posin(1, :), (-0.9 * (foot_x / 2) / 100 + a_loc2_modified(1, :)));

    % Call saturationBlock for posouty
    posouty = saturationBlock((0.9 * ((foot_y / 2) / 100) + a_loc2_modified(2, :)), posin(2, :), (-0.9 * ((foot_x / 2) / 100) + a_loc2_modified(2, :)));

    % % Obtain stepFwd and stepLat from zeroOrderHold function using the current time (k)
    % stepFwd = zeroOrderHold(posoutx, i - 1, i, 0.3);
    % stepLat = zeroOrderHold(posouty, i - 1, i, 0.3);
    % 
    % % Obtain stepFwd and stepLat from zeroOrderHold function using the current time (k)
    % stepFwd_1 = stepFwd *100;
    % stepLat_1 = stepLat *100;

%     if (rem(fix(i / 6), 2) == 0)
%         [footR, footL] = stateflowRL(stepFwd_1, stepLat_1, i, xL, yL, zL, xR, yR, zR, xrefL, yrefL, zrefL, xrefR, yrefR, zrefR, low, high); %right foot
% else
%         [footR, footL] = stateflowLR(stepFwd_1, stepLat_1, i, xL, yL, zL, xR, yR, zR, xrefL, yrefL, zrefL, xrefR, yrefR, zrefR, low, high); %left foot
%     end
end

function output = saturationBlock(input1, input2, input3)
    % Define lower and upper limits
    lower_limit = input3; % Define lower limit
    upper_limit = input1;  % Define upper limit

    % Calculate output
    output = min(upper_limit, max(lower_limit, input2));

    % % Ensure output type is integer and rounding mode is floor
    % output = floor(output);
end

% function output = zeroOrderHold(input, previousTime, currentTime, holdDuration)
%     persistent temp prevTime
% 
%     if isempty(temp) || previousTime ~= prevTime
%         temp = input;
%         prevTime = previousTime;
%     end
% 
%     if (currentTime - previousTime) >= holdDuration
%         output = input;
%     else
%         output = temp;
%     end
% end

== matlab function singlcontact_control_smc_lqr_mydimes_reaction/Walking Robot/smc+lqr+neuro1+reaction1/MATLAB Function ==
  data: smc_output input; blended_output output; lqr_output input; switch_flag input; transition_rate input
function blended_output = smooth_blend(smc_output, lqr_output, switch_flag, transition_rate)
    % Inputs:
    % smc_output: 3-element vector from SMC (e.g., [knee, hip_roll, hip_pitch])
    % lqr_output: 3-element vector from LQR (e.g., [knee, hip_roll, hip_pitch])
    % switch_flag: Binary signal indicating whether to use SMC (1) or LQR (0)
    % transition_rate: Rate of blending transition (0 to 1 range per step)
    
    % Initialize blended_output as the same size as input vectors
    blended_output = zeros(3, 1);

    % Loop through each joint control element
    for i = 1:3
        % Calculate smooth blend for each element
        blended_output(i) = (1 - transition_rate) * smc_output(i) + transition_rate * lqr_output(i);
    end
    
    % Adjust transition rate based on switch_flag
    if switch_flag == 1
        % When switch_flag is 1, stay closer to SMC output
        transition_rate = max(transition_rate - 0.05, 0);  % Adjust rate as needed
    else
        % When switch_flag is 0, move towards LQR output
        transition_rate = min(transition_rate + 0.05, 1);  % Adjust rate as needed
    end
end
